simulink model "project_part3_simulation"  (R2024a)
settings: Solver=VariableStepAuto  StartTime=0.0  StopTime=3  RelTol=1e-3
undefined symbols (not defined in the file): b, J, K, Kc, L, Lt, Nbar, R
settings Model: Creator=Harish  LastModifiedBy=Harish

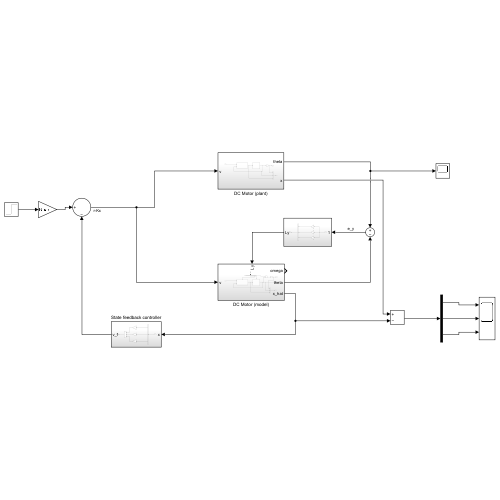
[thumbnail: Simulink's stored preview of the top-level diagram]
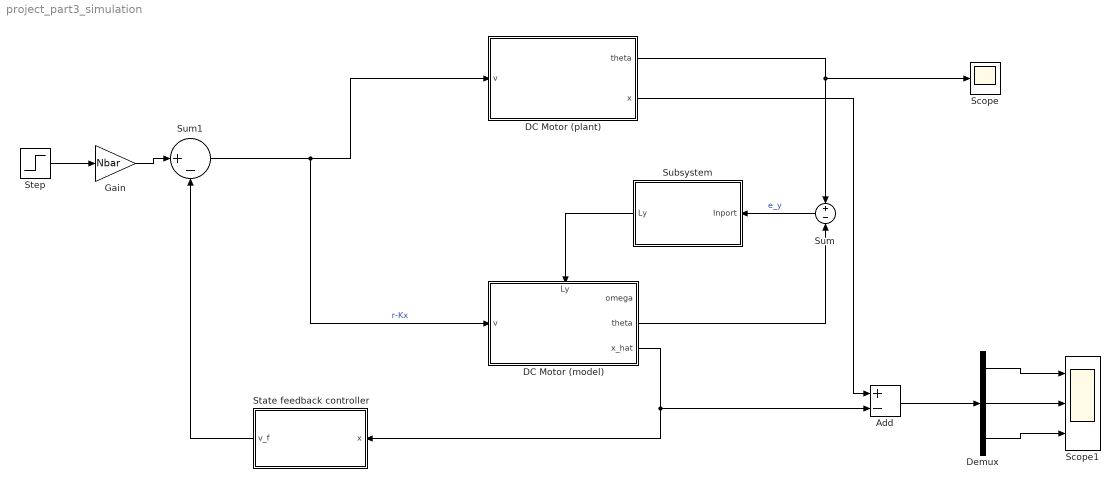
== system project_part3_simulation ==
  Add : Sum  Inputs=+-
  DC Motor (model) : Subsystem
      settings: PortSchema="{\"entries\":[{\"content\":{\"sides\":[{\"content\":{\"connectorIds\":[\"In1\"]},\"type\":\"ConnectorPlacement.EquallySpacedRectSide\",\"uuid\":\"754869d3-34ac-4187-a265-18eb04dc79de\"},{\"content\":{\"connectorIds\":[\"Out1\",\"Out2\",\"Out3\"],\"side\":\"RIGHT\"},\"type\":\"ConnectorPlacement.EquallySpacedRectSide\",\"uuid\":\"bca57fbc-c533-45e4-98a7-3f2b50abc1c8\"},{\"content\":{\"connectorIds\":[\"In2\"],\"side\":\"TOP\"},\"type\":\"ConnectorPlacement.EquallySpacedRectSide\",\"uuid\":\"40f17030-cb20-4681-97be-7a3ba1130cc0\"}]},\"type\":\"ConnectorPlacement.EquallySpacedConnector\",\"uuid\":\"f4c7f9b1-9417-4307-8b3e-4fda2b8e6c9d\"}],\"packageUris\":[\"http://schema.mathworks.com/mf0/Connector/R2020b\"],\"version\":\"1.0\"}"
  DC Motor (plant) : Subsystem
  Demux : Demux  Outputs=3
  Gain : Gain  Gain=Nbar
  Scope : Scope
  Scope1 : Scope  NumInputPorts=3
  State feedback controller : Subsystem
  Step : Step  SampleTime=0
  Subsystem : Subsystem
  Sum : Sum  Inputs=+-
  Sum1 : Sum  Inputs=|+-
  wires:
  DC Motor (plant)/1(theta) -> Sum/1, Scope/1
  DC Motor (model)/2(theta) -> Sum/2
  Sum/1 -> Subsystem/1(Inport)  "e_y"
  Subsystem/1(Ly) -> DC Motor (model)/2(Ly)
  Step/1 -> Gain/1
  State feedback controller/1(v_f) -> Sum1/2
  Sum1/1 -> DC Motor (model)/1(v), DC Motor (plant)/1(v)  "r-Kx"
  Gain/1 -> Sum1/1
  DC Motor (model)/3(x_hat) -> State feedback controller/1(x), Add/2
  DC Motor (plant)/2(x) -> Add/1
  Add/1 -> Demux/1
  Demux/1 -> Scope1/1
  Demux/2 -> Scope1/2
  Demux/3 -> Scope1/3

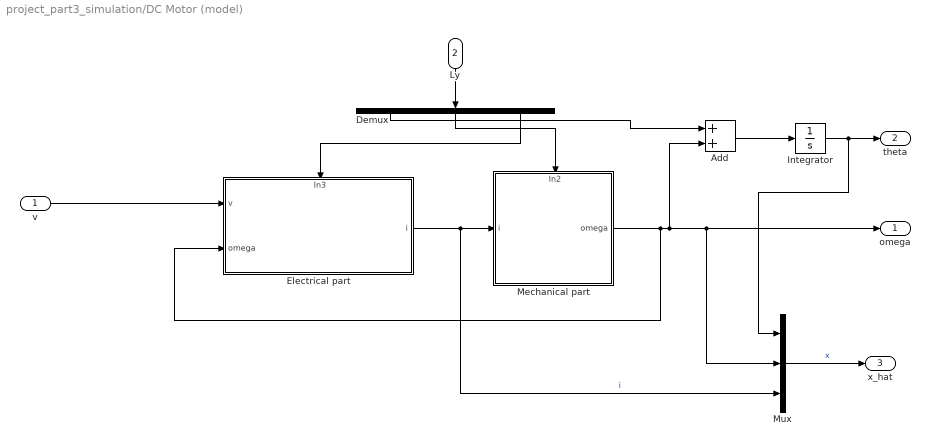
== system project_part3_simulation/DC Motor (model) ==
  v : Inport
  Ly : Inport  Port=2
  Add : Sum
  Demux : Demux  Outputs=3
  "Electrical part " : Subsystem
      settings: PortSchema="{\"entries\":[{\"content\":{\"sides\":[{\"content\":{\"connectorIds\":[\"In1\",\"In2\"]},\"type\":\"ConnectorPlacement.EquallySpacedRectSide\",\"uuid\":\"9733f2b1-a6a4-49fa-9220-2dece6bea88d\"},{\"content\":{\"connectorIds\":[\"Out1\"],\"side\":\"RIGHT\"},\"type\":\"ConnectorPlacement.EquallySpacedRectSide\",\"uuid\":\"d773a01d-026d-4b88-b527-91e3156ab25a\"},{\"content\":{\"connectorIds\":[\"In3\"],\"side\":\"TOP\"},\"type\":\"ConnectorPlacement.EquallySpacedRectSide\",\"uuid\":\"1b7c003c-33d0-43a8-b640-62c6bb83d28e\"}]},\"type\":\"ConnectorPlacement.EquallySpacedConnector\",\"uuid\":\"640833e1-1619-4539-ac9a-dd3b690716ef\"}],\"packageUris\":[\"http://schema.mathworks.com/mf0/Connector/R2020b\"],\"version\":\"1.0\"}"
  Integrator : Integrator
  Mechanical part : Subsystem
      settings: PortSchema="{\"entries\":[{\"content\":{\"sides\":[{\"content\":{\"connectorIds\":[\"In1\"]},\"type\":\"ConnectorPlacement.EquallySpacedRectSide\",\"uuid\":\"28580cc3-edec-43ce-9992-595d778b55e2\"},{\"content\":{\"connectorIds\":[\"Out1\"],\"side\":\"RIGHT\"},\"type\":\"ConnectorPlacement.EquallySpacedRectSide\",\"uuid\":\"5ed3f43d-89e0-4513-811a-de6e0a4508e3\"},{\"content\":{\"connectorIds\":[\"In2\"],\"side\":\"TOP\"},\"type\":\"ConnectorPlacement.EquallySpacedRectSide\",\"uuid\":\"8bac300d-be84-44c7-af02-52974f09fd5e\"}]},\"type\":\"ConnectorPlacement.EquallySpacedConnector\",\"uuid\":\"b610ff99-a488-485c-8b99-6a13c9745cb5\"}],\"packageUris\":[\"http://schema.mathworks.com/mf0/Connector/R2020b\"],\"version\":\"1.0\"}"
  Mux : Mux  Inputs=3
  omega : Outport
  theta : Outport  Port=2
  x_hat : Outport  Port=3
  wires:
  Mux/1 -> x_hat/1  "x"
  Integrator/1 -> Mux/1, theta/1
  v/1 -> "Electrical part "/1(v)
  Mechanical part/1(omega) -> "Electrical part "/2(omega), Add/2, Mux/2, omega/1
  "Electrical part "/1(i) -> Mux/3, Mechanical part/1(i)  "i"
  Ly/1 -> Demux/1
  Demux/3 -> "Electrical part "/3(In3)
  Demux/2 -> Mechanical part/2(In2)
  Demux/1 -> Add/1
  Add/1 -> Integrator/1

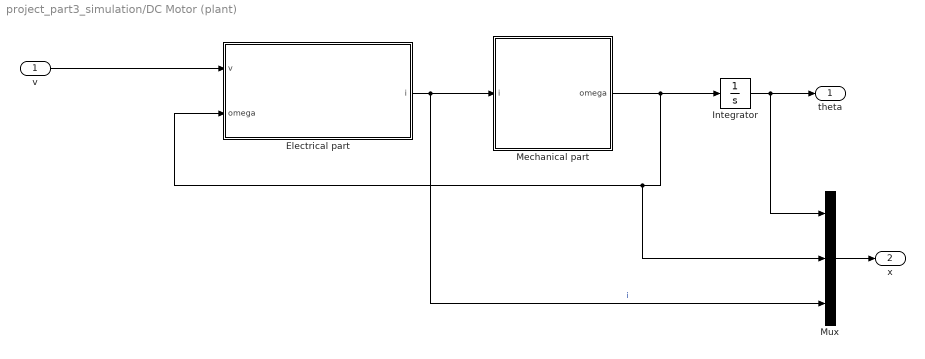
== system project_part3_simulation/DC Motor (plant) ==
  v : Inport
  "Electrical part " : Subsystem
  Integrator : Integrator  InitialCondition=0.5
  Mechanical part : Subsystem
  Mux : Mux  Inputs=3
  theta : Outport
  x : Outport  Port=2
  wires:
  "Electrical part "/1(i) -> Mux/3, Mechanical part/1(i)  "i"
  Mechanical part/1(omega) -> Integrator/1, Mux/2, "Electrical part "/2(omega)
  v/1 -> "Electrical part "/1(v)
  Integrator/1 -> Mux/1, theta/1
  Mux/1 -> x/1

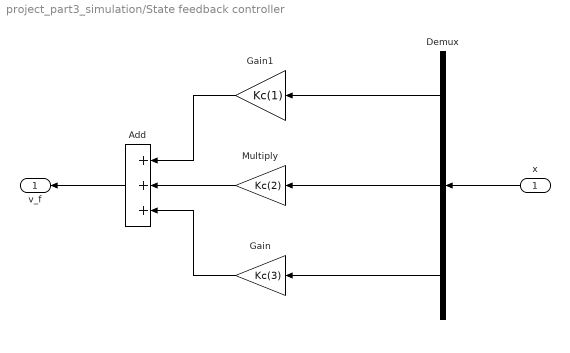
== system project_part3_simulation/State feedback controller ==
  x : Inport
  Add : Sum  Inputs=+++
  Demux : Demux  Outputs=3
  Gain : Gain  Gain=Kc(3)
  Gain1 : Gain  Gain=Kc(1)
  Multiply : Gain  Gain=Kc(2)
  v_f : Outport
  wires:
  Add/1 -> v_f/1
  x/1 -> Demux/1
  Demux/1 -> Gain1/1
  Demux/2 -> Multiply/1
  Demux/3 -> Gain/1
  Multiply/1 -> Add/2
  Gain1/1 -> Add/1
  Gain/1 -> Add/3

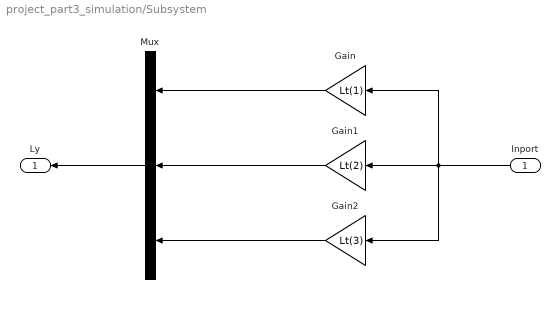
== system project_part3_simulation/Subsystem ==
  Inport : Inport
  Gain : Gain  Gain=Lt(1)
  Gain1 : Gain  Gain=Lt(2)
  Gain2 : Gain  Gain=Lt(3)
  Mux : Mux  Inputs=3
  Ly : Outport
  wires:
  Inport/1 -> Gain/1, Gain1/1, Gain2/1
  Gain/1 -> Mux/1
  Gain1/1 -> Mux/2
  Gain2/1 -> Mux/3
  Mux/1 -> Ly/1

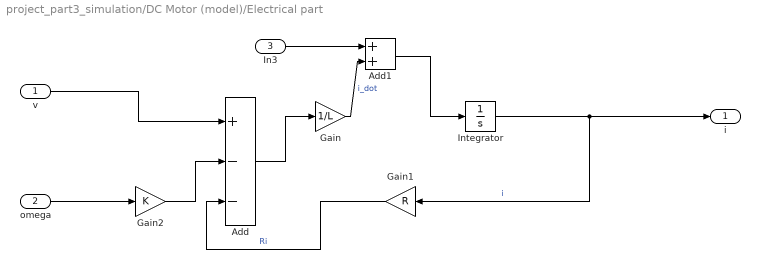
== system project_part3_simulation/DC Motor (model)/Electrical part  ==
  v : Inport
  omega : Inport  Port=2
  In3 : Inport  Port=3
  Add : Sum  Inputs=+--
  Add1 : Sum
  Gain : Gain  Gain=1/L
  Gain1 : Gain  Gain=R
  Gain2 : Gain  Gain=K
  Integrator : Integrator
  i : Outport
  wires:
  omega/1 -> Gain2/1
  Gain2/1 -> Add/2
  v/1 -> Add/1
  Gain1/1 -> Add/3  "Ri"
  Integrator/1 -> Gain1/1, i/1  "i"
  Add/1 -> Gain/1
  In3/1 -> Add1/1
  Gain/1 -> Add1/2  "i_dot"
  Add1/1 -> Integrator/1

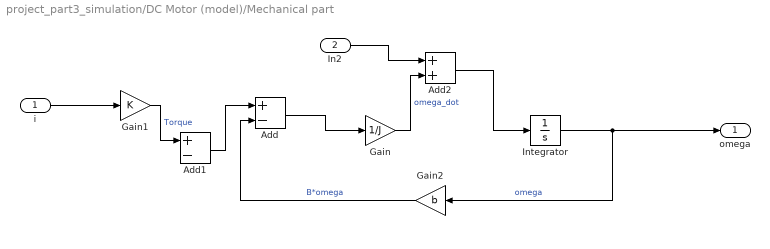
== system project_part3_simulation/DC Motor (model)/Mechanical part ==
  i : Inport
  In2 : Inport  Port=2
  Add : Sum  Inputs=+-
  Add1 : Sum  Inputs=+-
  Add2 : Sum
  Gain : Gain  Gain=1/J
  Gain1 : Gain  Gain=K
  Gain2 : Gain  Gain=b
  Integrator : Integrator
  omega : Outport
  wires:
  Add1/1 -> Add/1
  Gain1/1 -> Add1/1  "Torque"
  i/1 -> Gain1/1
  Gain2/1 -> Add/2  "B*omega"
  Integrator/1 -> Gain2/1, omega/1  "omega"
  Add/1 -> Gain/1
  In2/1 -> Add2/1
  Gain/1 -> Add2/2  "omega_dot"
  Add2/1 -> Integrator/1

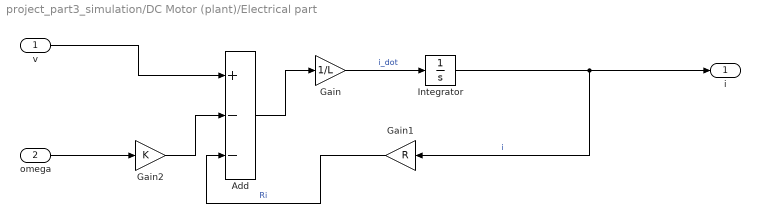
== system project_part3_simulation/DC Motor (plant)/Electrical part  ==
  v : Inport
  omega : Inport  Port=2
  Add : Sum  Inputs=+--
  Gain : Gain  Gain=1/L
  Gain1 : Gain  Gain=R
  Gain2 : Gain  Gain=K
  Integrator : Integrator  InitialCondition=0.5
  i : Outport
  wires:
  Add/1 -> Gain/1
  Integrator/1 -> i/1, Gain1/1  "i"
  Gain1/1 -> Add/3  "Ri"
  v/1 -> Add/1
  Gain2/1 -> Add/2
  Gain/1 -> Integrator/1  "i_dot"
  omega/1 -> Gain2/1

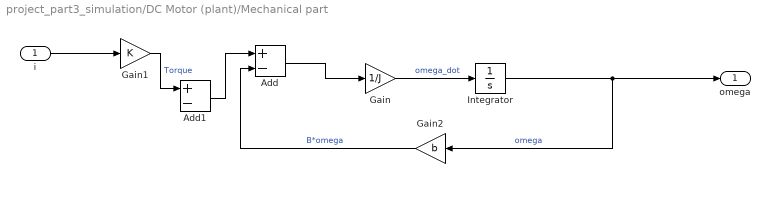
== system project_part3_simulation/DC Motor (plant)/Mechanical part ==
  i : Inport
  Add : Sum  Inputs=+-
  Add1 : Sum  Inputs=+-
  Gain : Gain  Gain=1/J
  Gain1 : Gain  Gain=K
  Gain2 : Gain  Gain=b
  Integrator : Integrator  InitialCondition=0.05
  omega : Outport
  wires:
  Add/1 -> Gain/1
  Integrator/1 -> omega/1, Gain2/1  "omega"
  Gain2/1 -> Add/2  "B*omega"
  i/1 -> Gain1/1
  Gain/1 -> Integrator/1  "omega_dot"
  Gain1/1 -> Add1/1  "Torque"
  Add1/1 -> Add/1
